simulink model "DT_SigmaDelta"  (Simulink 7.9)
settings: Solver=VariableStepDiscrete  StartTime=0.0  StopTime=1  RelTol=1e-6
PreLoadFcn:
  | load one_stage.mat
undefined symbols (not defined in the file or in its folder): DiscIntNeverNeededParam
libraries: dspmlti4 x21, simulink x3, dspvision x1
(part 1 of 13)
settings Model: Creator=abehbood  LastModifiedBy=Arnaldi Isacco
settings SolverCC: ConsecutiveZCsStepRelTol=128*eps  ZeroCrossControl=DisableAll
settings DataIOCC: LimitDataPoints=off  SaveFormat=StructureWithTime  SaveOutput=off  SaveTime=off
settings OptimizationCC: InitFltsAndDblsToZero=on
settings DebuggingCC: AlgebraicLoopMsg=none  SaveWithParameterizedLinksMsg=none  SignalResolutionControl=TryResolveAllWithWarning  FcnCallInpInsideContextMsg=Use local settings  StrictBusMsg=Warning
settings SFSimCC: SimParseCustomCode=off
settings GRTTargetCC: TargetFcnLib=ansi_tfl_tmw.mat  CombineOutputUpdateFcns=off  GRTInterface=on
settings ConfigurationSet: Description=SimMechanics 2G

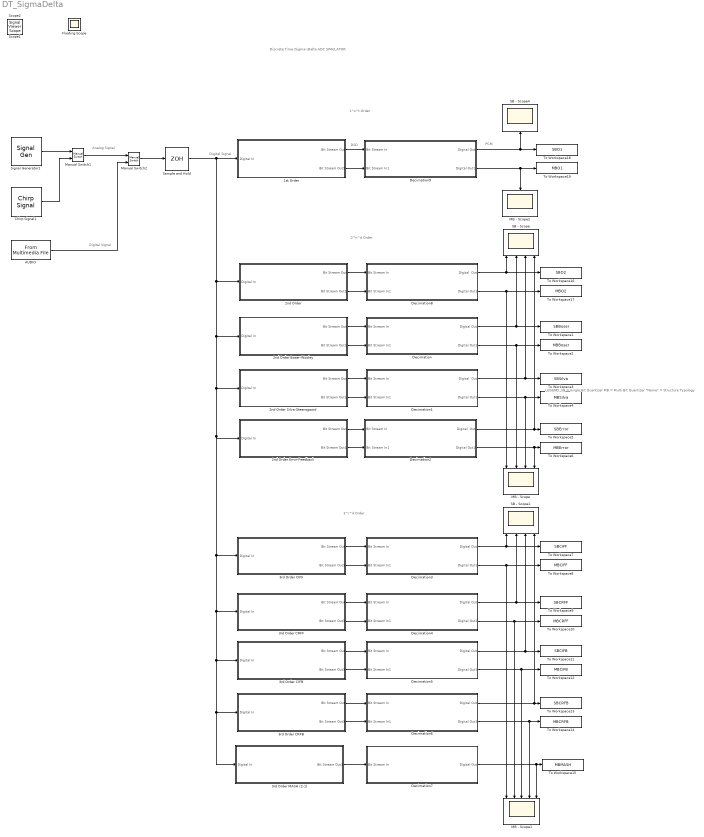
== system DT_SigmaDelta ==
  note: Discrete Time
      | \Sigma-\Delta ADC
      | SIMULATOR
  note: Digital Signal
  note: LEGEND:
      |
      | SB = Single Bit Quantizer
      |
      | MB = Multi Bit Quantizer
      |
      | "Name" = Structure Typology
  note: 2^n^d Order
  note: 3^r^d Order
  note: 1^s^t Order
  note: Analog Signal
  note: Digital Signal
  note: DSD
  note: PCM
  1st Order : Subsystem
  "2nd Order  " : Subsystem
  2nd Order Boser-Wooley : Subsystem
  2nd Order Error-Feedback : Subsystem
  "2nd Order Silva-Steensgaard " : Subsystem
  3rd Order CIFB : Subsystem
  3rd Order CIFF : Subsystem
  3rd Order CRFB : Subsystem
  3rd Order CRFF : Subsystem
  3rd Order MASH (2-1) : Subsystem
  AUDIO : dspvision/From Multimedia File  inputFilename=.\AudioSample.wav  loop=on  numPlays=inf  outputStreams=Audio only  videoDataType=single  audioDataType=double  inheritSampleTime=on  userDefinedSampleTime=1/30  noAudioOutput=off  isIntensityVideo=off  fourcc=RGB  colorVideoFormat=One multidimensional signal  outputEOF=off  dataOrg=Column-major  audioFrameSize=1  computeAudioFrameSize=off  outSamplingMode=Sample based
  Chirp Signal1 : simulink/Sources/Chirp Signal  f1=0.1  T=24/3000  f2=10000
  Decimation : Subsystem
  Decimation1 : Subsystem
  Decimation2 : Subsystem
  Decimation3 : Subsystem
  Decimation4 : Subsystem
  Decimation5 : Subsystem
  Decimation6 : Subsystem
  Decimation7 : Subsystem
  Decimation8 : Subsystem
  Decimation9 : Subsystem
  MB - Scope : Scope  NumInputPorts=4
      settings: TimeRange=0.008  YMin=-1.25~-1~-1~-5  YMax=1~1~1~5  SaveName=ScopeData2
  MB - Scope1 : Scope  NumInputPorts=5
      settings: TimeRange=0.008  YMin=-1.25~-1.25~-0.7~-0.75~-5  YMax=1.25~1.25~0.7~0.75~5  SaveName=ScopeData3
  MB - Scope2 : Scope
      settings: TimeRange=0.008  YMin=-1.25  YMax=1  SaveName=ScopeData6
  Manual Switch1 : simulink/Signal Routing/Manual Switch  sw=1  action=0  varsize=off
  Manual Switch2 : simulink/Signal Routing/Manual Switch  sw=1  action=0  varsize=off
  SB - Scope : Scope  NumInputPorts=4
      settings: TimeRange=0.008  YMin=-0.015~-0.01~-0.01~-0.015  YMax=0.015~0.0075~0.0125~0.015
  SB - Scope1 : Scope  NumInputPorts=4
      settings: TimeRange=0.008  YMin=-1.25~-0.8~-0.8~-0.75  YMax=1.25~0.8~0.8~0.75  SaveName=ScopeData4
  SB - Scope4 : Scope
      settings: TimeRange=0.008  YMin=-0.75  YMax=0.75  SaveName=ScopeData8
  Sample and Hold : ZeroOrderHold  SampleTime=1/(48e3*64)
  Signal Generator1 : SignalGenerator  Frequency=6283  Units=rad/sec
  To Workspace1 : ToWorkspace  VariableName=SBBoser  SampleTime=-1
  To Workspace10 : ToWorkspace  VariableName=MBCRFF  SampleTime=-1
  To Workspace11 : ToWorkspace  VariableName=SBCIFB  SampleTime=-1
  To Workspace12 : ToWorkspace  VariableName=MBCIFB  SampleTime=-1
  To Workspace13 : ToWorkspace  VariableName=SBCRFB  SampleTime=-1
  To Workspace14 : ToWorkspace  VariableName=MBCRFB  SampleTime=-1
  To Workspace15 : ToWorkspace  VariableName=MBMASH  SampleTime=-1
  To Workspace16 : ToWorkspace  VariableName=SBO2  SampleTime=-1
  To Workspace17 : ToWorkspace  VariableName=MBO2  SampleTime=-1
  To Workspace18 : ToWorkspace  VariableName=SBO1  SampleTime=-1
  To Workspace19 : ToWorkspace  VariableName=MBO1  SampleTime=-1
  To Workspace2 : ToWorkspace  VariableName=MBBoser  SampleTime=-1
  To Workspace3 : ToWorkspace  VariableName=SBSilva  SampleTime=-1
  To Workspace4 : ToWorkspace  VariableName=MBSilva  SampleTime=-1
  To Workspace5 : ToWorkspace  VariableName=SBError  SampleTime=-1
  To Workspace6 : ToWorkspace  VariableName=MBError  SampleTime=-1
  To Workspace7 : ToWorkspace  VariableName=SBCIFF  SampleTime=-1
  To Workspace8 : ToWorkspace  VariableName=MBCIFF  SampleTime=-1
  To Workspace9 : ToWorkspace  VariableName=SBCRFF  SampleTime=-1
  Floating Scope : Scope
      settings: Floating=on  YMin=-1  YMax=1
  Scope1 : SignalViewerScope  IOType=viewer  RefreshTime=0.035000
  Scope2 : SignalViewerScope  IOType=viewer  RefreshTime=0.035000
  wires:
  Decimation/1(Digital Out) -> To Workspace1/1, SB - Scope/2
  Decimation/2(Digital Out1) -> To Workspace2/1, MB - Scope/2
  Decimation1/1(Digital  Out) -> To Workspace3/1, SB - Scope/3
  Decimation1/2(Digital Out1) -> To Workspace4/1, MB - Scope/3
  Decimation2/1(Digital  Out) -> To Workspace5/1, SB - Scope/4
  Decimation2/2(Digital Out1) -> To Workspace6/1, MB - Scope/4
  Sample and Hold/1 -> 1st Order/1("Digital In "), "2nd Order  "/1(Digital In), 2nd Order Boser-Wooley/1("Digital In "), "2nd Order Silva-Steensgaard "/1(Digital In), 2nd Order Error-Feedback/1(Digital In), 3rd Order CIFB/1("Digital In "), 3rd Order CRFB/1("Digital In "), 3rd Order MASH (2-1)/1("Digital In "), 3rd Order CRFF/1(Digital In), 3rd Order CIFF/1(Digital In)
  2nd Order Boser-Wooley/2(Bit Stream Out1) -> Decimation/2(Bit Stream In1)
  2nd Order Boser-Wooley/1(Bit Stream Out) -> Decimation/1(Bit Stream In)
  "2nd Order Silva-Steensgaard "/1(Bit Stream Out) -> Decimation1/1(Bit Stream In)
  "2nd Order Silva-Steensgaard "/2(Bit Stream Out1) -> Decimation1/2(Bit Stream In1)
  2nd Order Error-Feedback/1(Bit Stream Out) -> Decimation2/1(Bit Stream In)
  2nd Order Error-Feedback/2(Bit Stream Out1) -> Decimation2/2(Bit Stream In1)
  Decimation6/1(Digital Out) -> To Workspace13/1, SB - Scope1/4
  Decimation6/2(Digital Out1) -> To Workspace14/1, MB - Scope1/4
  3rd Order CRFB/1(Bit Stream Out) -> Decimation6/1(Bit Stream In)
  3rd Order CRFB/2(Bit Stream Out1) -> Decimation6/2(Bit Stream In1)
  Decimation7/1(Digital Out) -> To Workspace15/1, MB - Scope1/5
  3rd Order MASH (2-1)/1(Bit Stream Out1) -> Decimation7/1(Bit Stream In)
  Decimation5/1(Digital Out) -> To Workspace11/1, SB - Scope1/3
  Decimation5/2(Digital Out1) -> To Workspace12/1, MB - Scope1/3
  Decimation4/1(Digital Out) -> To Workspace9/1, SB - Scope1/2
  Decimation4/2(Digital Out1) -> To Workspace10/1, MB - Scope1/2
  Decimation3/1(Digital Out) -> To Workspace7/1, SB - Scope1/1
  Decimation3/2(Digital Out1) -> To Workspace8/1, MB - Scope1/1
  3rd Order CIFF/1(Bit Stream Out) -> Decimation3/1(Bit Stream In)
  3rd Order CIFF/2(Bit Stream Out1) -> Decimation3/2(Bit Stream In1)
  3rd Order CIFB/1(Bit Stream Out) -> Decimation5/1(Bit Stream In)
  3rd Order CIFB/2(Bit Stream Out1) -> Decimation5/2(Bit Stream In1)
  "2nd Order  "/1(Bit Stream Out) -> Decimation8/1(Bit Stream In)
  "2nd Order  "/2(Bit Stream Out1) -> Decimation8/2(Bit Stream In1)
  Decimation8/1(Digital  Out) -> SB - Scope/1, To Workspace16/1
  Decimation8/2(Digital Out1) -> MB - Scope/1, To Workspace17/1
  Decimation9/1(Digital Out) -> To Workspace18/1, SB - Scope4/1
  1st Order/1(" Bit Stream Out") -> Decimation9/1(Bit Stream In)
  1st Order/2(" Bit Stream Out1") -> Decimation9/2(Bit Stream In1)
  Decimation9/2(Digital Out1) -> MB - Scope2/1, To Workspace19/1
  Signal Generator1/1 -> Manual Switch1/1
  Chirp Signal1/1 -> Manual Switch1/2
  Manual Switch1/1 -> Manual Switch2/1
  Manual Switch2/1 -> Sample and Hold/1
  AUDIO/1 -> Manual Switch2/2
  3rd Order CRFF/1(Bit Stream Out) -> Decimation4/1(Bit Stream In)
  3rd Order CRFF/2(Bit Stream Out1) -> Decimation4/2(Bit Stream In1)

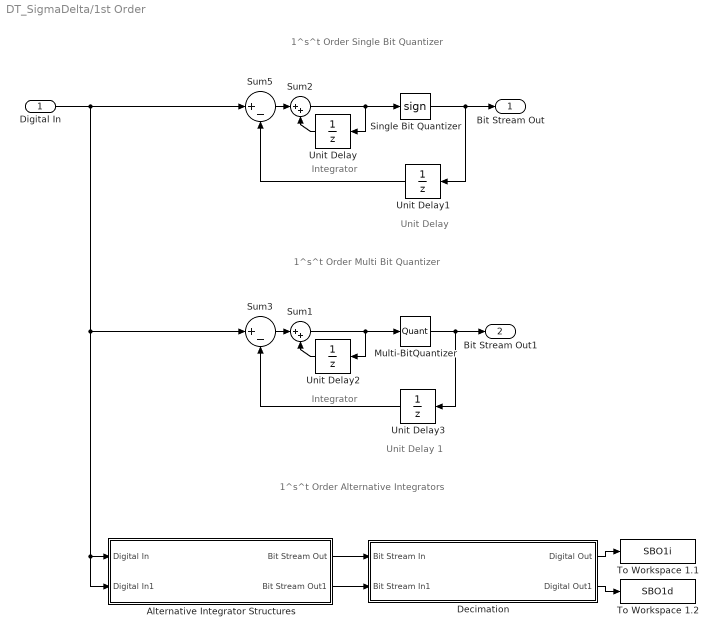
== system DT_SigmaDelta/1st Order ==
  note: 1^s^t Order Single Bit Quantizer
  note: 1^s^t Order Multi Bit Quantizer
  note: 1^s^t Order Alternative Integrators
  note: Integrator
  note: Integrator
  note: Unit Delay 1
  note: Unit Delay
  "Digital In " : Inport
  Alternative Integrator Structures : Subsystem
  Decimation : Subsystem
  Multi-BitQuantizer : Quantizer  QuantizationInterval=0.14  SampleTime=1/(48e3*64)
  Single Bit Quantizer : Signum  SampleTime=1/(48e3*64)
  Sum1 : Sum  Inputs=|++
  Sum2 : Sum  Inputs=|++
  Sum3 : Sum  Inputs=|+-  AccumDataTypeStr=double  SampleTime=1/(48e3*64)
  Sum5 : Sum  Inputs=|+-  AccumDataTypeStr=double  SampleTime=1/(48e3*64)
  To Workspace 1.1 : ToWorkspace  VariableName=SBO1i  SampleTime=-1
  To Workspace 1.2 : ToWorkspace  VariableName=SBO1d  SampleTime=-1
  Unit Delay{,1..3} (4 alike) : UnitDelay  SampleTime=1/(48e3*64)
  " Bit Stream Out" : Outport  OutDataTypeStr=double
  " Bit Stream Out1" : Outport  Port=2  OutDataTypeStr=double
  wires:
  "Digital In "/1 -> Sum5/1, Sum3/1, Alternative Integrator Structures/1(Digital In), Alternative Integrator Structures/2(Digital In1)
  Sum5/1 -> Sum2/1
  Unit Delay/1 -> Sum2/2
  Unit Delay1/1 -> Sum5/2
  Sum2/1 -> Unit Delay/1, Single Bit Quantizer/1
  Single Bit Quantizer/1 -> " Bit Stream Out"/1, Unit Delay1/1
  Sum3/1 -> Sum1/1
  Unit Delay2/1 -> Sum1/2
  Unit Delay3/1 -> Sum3/2
  Sum1/1 -> Unit Delay2/1, Multi-BitQuantizer/1
  Multi-BitQuantizer/1 -> Unit Delay3/1, " Bit Stream Out1"/1
  Decimation/1(Digital Out) -> To Workspace 1.1/1
  Alternative Integrator Structures/1(Bit Stream Out) -> Decimation/1(Bit Stream In)
  Alternative Integrator Structures/2(Bit Stream Out1) -> Decimation/2(Bit Stream In1)
  Decimation/2(Digital Out1) -> To Workspace 1.2/1

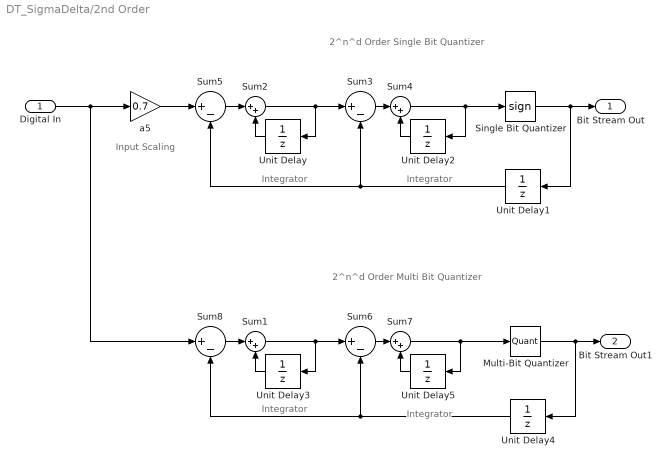
== system DT_SigmaDelta/2nd Order   ==
  note: 2^n^d Order Single Bit Quantizer
  note: 2^n^d Order Multi Bit Quantizer
  note: Input Scaling
  note: Integrator
  note: Integrator
  note: Integrator
  note: Integrator
  Digital In : Inport
  Multi-Bit Quantizer : Quantizer  QuantizationInterval=0.15  SampleTime=1/(48e3*64)
  Single Bit Quantizer : Signum  SampleTime=1/(48e3*64)
  Sum{1..2,4,7} (4 alike) : Sum  Inputs=|++  SampleTime=1/(48e3*64)
  Sum{3,5..6,8} (4 alike) : Sum  Inputs=|+-  AccumDataTypeStr=double  SampleTime=1/(48e3*64)
  Unit Delay{,1..5} (6 alike) : UnitDelay  SampleTime=1/(48e3*64)
  a5 : Gain  Gain=0.7  SampleTime=1/(48e3*64)
  Bit Stream Out : Outport  OutDataTypeStr=double
  Bit Stream Out1 : Outport  Port=2  OutDataTypeStr=double
  wires:
  Digital In/1 -> a5/1, Sum8/1
  Single Bit Quantizer/1 -> Bit Stream Out/1, Unit Delay1/1
  Multi-Bit Quantizer/1 -> Bit Stream Out1/1, Unit Delay4/1
  Sum8/1 -> Sum1/1
  Sum6/1 -> Sum7/1
  Unit Delay3/1 -> Sum1/2
  Sum1/1 -> Unit Delay3/1, Sum6/1
  Sum5/1 -> Sum2/1
  Unit Delay/1 -> Sum2/2
  Sum2/1 -> Sum3/1, Unit Delay/1
  Sum3/1 -> Sum4/1
  a5/1 -> Sum5/1
  Unit Delay2/1 -> Sum4/2
  Sum4/1 -> Unit Delay2/1, Single Bit Quantizer/1
  Unit Delay1/1 -> Sum5/2, Sum3/2
  Unit Delay5/1 -> Sum7/2
  Sum7/1 -> Unit Delay5/1, Multi-Bit Quantizer/1
  Unit Delay4/1 -> Sum8/2, Sum6/2

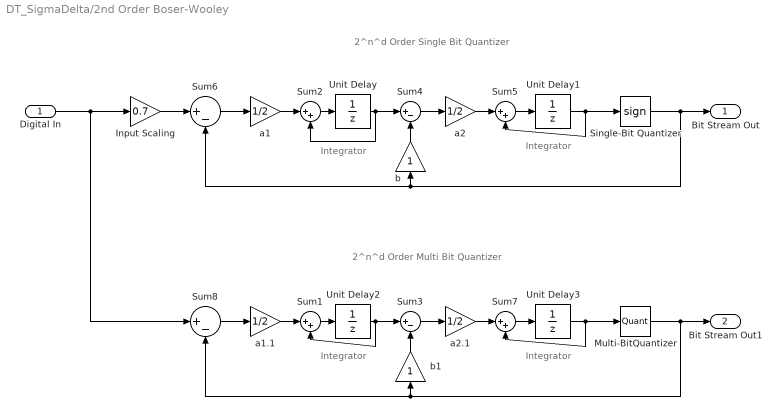
== system DT_SigmaDelta/2nd Order Boser-Wooley ==
  note: 2^n^d Order Single Bit Quantizer
  note: 2^n^d Order Multi Bit Quantizer
  note: Integrator
  note: Integrator
  note: Integrator
  note: Integrator
  "Digital In " : Inport
  Input Scaling : Gain  Gain=0.7  SampleTime=1/(48e3*64)
  Multi-BitQuantizer : Quantizer  QuantizationInterval=0.15  SampleTime=1/(48e3*64)
  Single-Bit Quantizer : Signum  SampleTime=1/(48e3*64)
  Sum{1..2,5,7} (4 alike) : Sum  Inputs=|++  SampleTime=1/(48e3*64)
  Sum3 : Sum  Inputs=|+-  SampleTime=1/(48e3*64)
  Sum4 : Sum  Inputs=|+-  SampleTime=1/(48e3*64)
  Sum6 : Sum  Inputs=|+-  AccumDataTypeStr=double  SampleTime=1/(48e3*64)
  Sum8 : Sum  Inputs=|+-  AccumDataTypeStr=double  SampleTime=1/(48e3*64)
  Unit Delay{,1..3} (4 alike) : UnitDelay  SampleTime=1/(48e3*64)
  a1 : Gain  Gain=1/2  SampleTime=1/(48e3*64)
  a1.1 : Gain  Gain=1/2  SampleTime=1/(48e3*64)
  a2 : Gain  Gain=1/2  SampleTime=1/(48e3*64)
  a2.1 : Gain  Gain=1/2  SampleTime=1/(48e3*64)
  b : Gain  SampleTime=1/(48e3*64)
  b1 : Gain  SampleTime=1/(48e3*64)
  Bit Stream Out : Outport  OutDataTypeStr=double
  Bit Stream Out1 : Outport  Port=2  OutDataTypeStr=double
  wires:
  "Digital In "/1 -> Input Scaling/1, Sum8/1
  Single-Bit Quantizer/1 -> b/1, Sum6/2, Bit Stream Out/1
  b/1 -> Sum4/2
  Sum5/1 -> Unit Delay1/1
  Sum6/1 -> a1/1
  Sum4/1 -> a2/1
  Unit Delay1/1 -> Single-Bit Quantizer/1, Sum5/2
  a2/1 -> Sum5/1
  a1/1 -> Sum2/1
  Unit Delay/1 -> Sum4/1, Sum2/2
  Sum2/1 -> Unit Delay/1
  Input Scaling/1 -> Sum6/1
  Multi-BitQuantizer/1 -> Bit Stream Out1/1, Sum8/2, b1/1
  b1/1 -> Sum3/2
  Sum7/1 -> Unit Delay3/1
  Sum8/1 -> a1.1/1
  Sum3/1 -> a2.1/1
  Unit Delay3/1 -> Sum7/2, Multi-BitQuantizer/1
  a2.1/1 -> Sum7/1
  a1.1/1 -> Sum1/1
  Unit Delay2/1 -> Sum1/2, Sum3/1
  Sum1/1 -> Unit Delay2/1

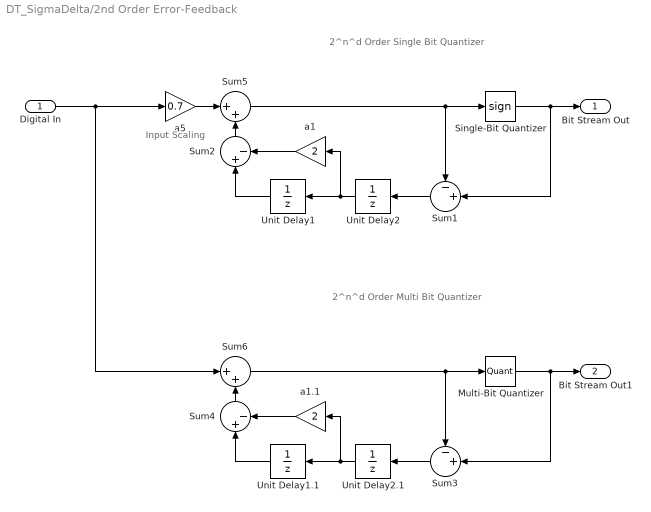
== system DT_SigmaDelta/2nd Order Error-Feedback ==
  note: Input Scaling
  note: 2^n^d Order Multi Bit Quantizer
  note: 2^n^d Order Single Bit Quantizer
  Digital In : Inport
  Multi-Bit Quantizer : Quantizer  QuantizationInterval=0.15  SampleTime=1/(48e3*64)
  Single-Bit Quantizer : Signum  SampleTime=1/(48e3*64)
  Sum1 : Sum  Inputs=-+|  AccumDataTypeStr=double  SampleTime=1/(48e3*64)
  Sum2 : Sum  Inputs=|+-  AccumDataTypeStr=double  SampleTime=1/(48e3*64)
  Sum3 : Sum  Inputs=-+|  AccumDataTypeStr=double  SampleTime=1/(48e3*64)
  Sum4 : Sum  Inputs=|+-  AccumDataTypeStr=double  SampleTime=1/(48e3*64)
  Sum5 : Sum  Inputs=|++  AccumDataTypeStr=double  SampleTime=1/(48e3*64)
  Sum6 : Sum  Inputs=|++  AccumDataTypeStr=double  SampleTime=1/(48e3*64)
  Unit Delay1 : UnitDelay  SampleTime=1/(48e3*64)
  Unit Delay1.1 : UnitDelay  SampleTime=1/(48e3*64)
  Unit Delay2 : UnitDelay  SampleTime=1/(48e3*64)
  Unit Delay2.1 : UnitDelay  SampleTime=1/(48e3*64)
  a1 : Gain  Gain=2  SampleTime=1/(48e3*64)
  a1.1 : Gain  Gain=2  SampleTime=1/(48e3*64)
  a5 : Gain  Gain=0.7  SampleTime=1/(48e3*64)
  Bit Stream Out : Outport  OutDataTypeStr=double
  Bit Stream Out1 : Outport  Port=2  OutDataTypeStr=double
  wires:
  Digital In/1 -> a5/1, Sum6/1
  Single-Bit Quantizer/1 -> Bit Stream Out/1, Sum1/2
  Unit Delay2/1 -> Unit Delay1/1, a1/1
  Unit Delay1/1 -> Sum2/1
  Sum2/1 -> Sum5/2
  a1/1 -> Sum2/2
  Sum5/1 -> Single-Bit Quantizer/1, Sum1/1
  Sum1/1 -> Unit Delay2/1
  a5/1 -> Sum5/1
  Multi-Bit Quantizer/1 -> Sum3/2, Bit Stream Out1/1
  Unit Delay2.1/1 -> a1.1/1, Unit Delay1.1/1
  Unit Delay1.1/1 -> Sum4/1
  Sum4/1 -> Sum6/2
  a1.1/1 -> Sum4/2
  Sum6/1 -> Sum3/1, Multi-Bit Quantizer/1
  Sum3/1 -> Unit Delay2.1/1

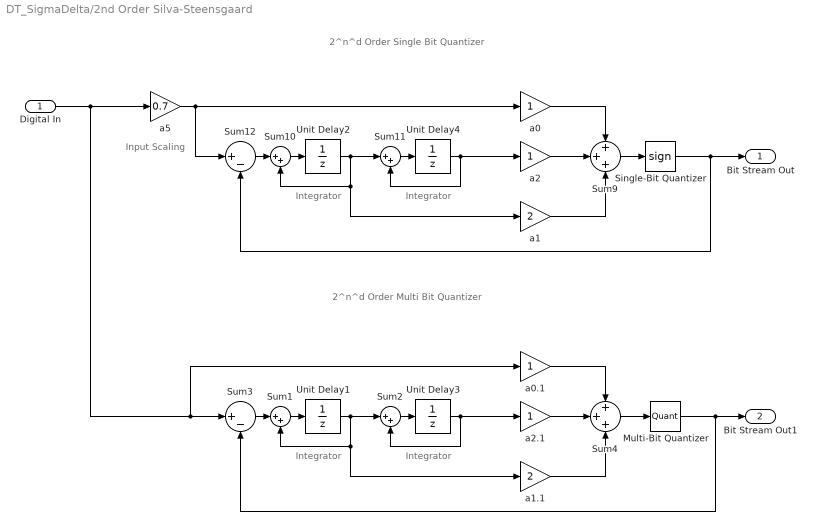
== system DT_SigmaDelta/2nd Order Silva-Steensgaard  ==
  note: 2^n^d Order Single Bit Quantizer
  note: 2^n^d Order Multi Bit Quantizer
  note: Input Scaling
  note: Integrator
  note: Integrator
  note: Integrator
  note: Integrator
  Digital In : Inport
  Multi-Bit Quantizer : Quantizer  QuantizationInterval=0.15  SampleTime=1/(48e3*64)
  Single-Bit Quantizer : Signum  SampleTime=1/(48e3*64)
  Sum{1..2,10..11} (4 alike) : Sum  Inputs=|++  SampleTime=1/(48e3*64)
  Sum12 : Sum  Inputs=|+-  AccumDataTypeStr=double  SampleTime=1/(48e3*64)
  Sum3 : Sum  Inputs=|+-  AccumDataTypeStr=double  SampleTime=1/(48e3*64)
  Sum4 : Sum  Inputs=+++  AccumDataTypeStr=double  SampleTime=1/(48e3*64)
  Sum9 : Sum  Inputs=+++  AccumDataTypeStr=double  SampleTime=1/(48e3*64)
  Unit Delay{1..4} (4 alike) : UnitDelay  SampleTime=1/(48e3*64)
  a0 : Gain  SampleTime=1/(48e3*64)
  a0.1 : Gain  SampleTime=1/(48e3*64)
  a1 : Gain  Gain=2  SampleTime=1/(48e3*64)
  a1.1 : Gain  Gain=2  SampleTime=1/(48e3*64)
  a2 : Gain  SampleTime=1/(48e3*64)
  a2.1 : Gain  SampleTime=1/(48e3*64)
  a5 : Gain  Gain=0.7  SampleTime=1/(48e3*64)
  Bit Stream Out : Outport  OutDataTypeStr=double
  Bit Stream Out1 : Outport  Port=2  OutDataTypeStr=double
  wires:
  Digital In/1 -> a5/1, Sum3/1, a0.1/1
  a5/1 -> a0/1, Sum12/1
  Unit Delay4/1 -> Sum11/2, a2/1
  Sum11/1 -> Unit Delay4/1
  Single-Bit Quantizer/1 -> Bit Stream Out/1, Sum12/2
  Sum12/1 -> Sum10/1
  Sum10/1 -> Unit Delay2/1
  Unit Delay2/1 -> Sum11/1, Sum10/2, a1/1
  a2/1 -> Sum9/2
  a0/1 -> Sum9/1
  a1/1 -> Sum9/3
  Sum9/1 -> Single-Bit Quantizer/1
  Unit Delay3/1 -> a2.1/1, Sum2/2
  Sum2/1 -> Unit Delay3/1
  Multi-Bit Quantizer/1 -> Sum3/2, Bit Stream Out1/1
  Sum3/1 -> Sum1/1
  Sum1/1 -> Unit Delay1/1
  Unit Delay1/1 -> a1.1/1, Sum1/2, Sum2/1
  a2.1/1 -> Sum4/2
  a0.1/1 -> Sum4/1
  a1.1/1 -> Sum4/3
  Sum4/1 -> Multi-Bit Quantizer/1

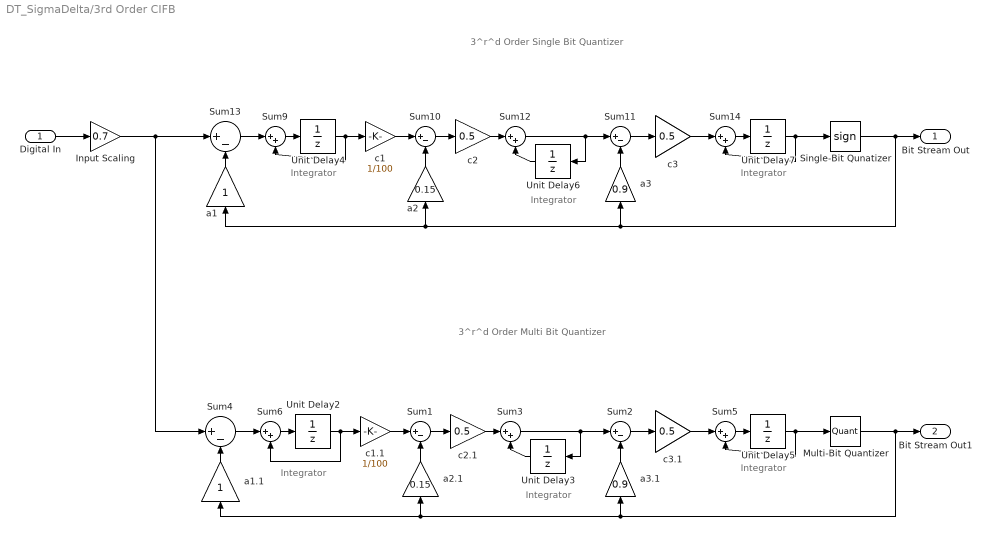
== system DT_SigmaDelta/3rd Order CIFB ==
  note: 3^r^d Order Single Bit Quantizer
  note: 3^r^d Order Multi Bit Quantizer
  note: Integrator
  note: Integrator
  note: Integrator
  note: Integrator
  note: Integrator
  note: Integrator
  "Digital In " : Inport
  Input Scaling : Gain  Gain=0.7  SampleTime=1/(48e3*64)
  Multi-Bit Quantizer : Quantizer  QuantizationInterval=0.15  SampleTime=1/(48e3*64)
  Single-Bit Qunatizer : Signum  SampleTime=1/(48e3*64)
  Sum{1..2,10..11} (4 alike) : Sum  Inputs=|+-
  Sum{3,5..6,9,12,14} (6 alike) : Sum  Inputs=|++  SampleTime=1/(48e3*64)
  Sum13 : Sum  Inputs=|+-  AccumDataTypeStr=double  SampleTime=1/(48e3*64)
  Sum4 : Sum  Inputs=|+-  AccumDataTypeStr=double  SampleTime=1/(48e3*64)
  Unit Delay{2..7} (6 alike) : UnitDelay  SampleTime=1/(48e3*64)
  a1 : Gain
  a1.1 : Gain
  a2 : Gain  Gain=0.15
  a2.1 : Gain  Gain=0.15
  a3 : Gain  Gain=0.9
  a3.1 : Gain  Gain=0.9
  c1 : Gain  Gain=1/100  SampleTime=1/(48e3*64)
  c1.1 : Gain  Gain=1/100  SampleTime=1/(48e3*64)
  c2 : Gain  Gain=0.5
  c2.1 : Gain  Gain=0.5
  c3 : Gain  Gain=0.5
  c3.1 : Gain  Gain=0.5
  Bit Stream Out : Outport  OutDataTypeStr=double
  Bit Stream Out1 : Outport  Port=2  OutDataTypeStr=double
  wires:
  c1/1 -> Sum10/1
  a2/1 -> Sum10/2
  "Digital In "/1 -> Input Scaling/1
  Single-Bit Qunatizer/1 -> a1/1, a2/1, a3/1, Bit Stream Out/1
  a3/1 -> Sum11/2
  a1/1 -> Sum13/2
  Sum13/1 -> Sum9/1
  Sum11/1 -> c3/1
  Sum10/1 -> c2/1
  Unit Delay6/1 -> Sum12/2
  Sum12/1 -> Sum11/1, Unit Delay6/1
  c2/1 -> Sum12/1
  c3/1 -> Sum14/1
  Input Scaling/1 -> Sum4/1, Sum13/1
  Multi-Bit Quantizer/1 -> a3.1/1, a2.1/1, a1.1/1, Bit Stream Out1/1
  a3.1/1 -> Sum2/2
  a1.1/1 -> Sum4/2
  Sum4/1 -> Sum6/1
  Sum2/1 -> c3.1/1
  Sum1/1 -> c2.1/1
  a2.1/1 -> Sum1/2
  c1.1/1 -> Sum1/1
  Unit Delay3/1 -> Sum3/2
  Sum3/1 -> Sum2/1, Unit Delay3/1
  c2.1/1 -> Sum3/1
  c3.1/1 -> Sum5/1
  Sum9/1 -> Unit Delay4/1
  Unit Delay4/1 -> Sum9/2, c1/1
  Sum14/1 -> Unit Delay7/1
  Unit Delay7/1 -> Single-Bit Qunatizer/1, Sum14/2
  Sum5/1 -> Unit Delay5/1
  Unit Delay5/1 -> Multi-Bit Quantizer/1, Sum5/2
  Sum6/1 -> Unit Delay2/1
  Unit Delay2/1 -> c1.1/1, Sum6/2

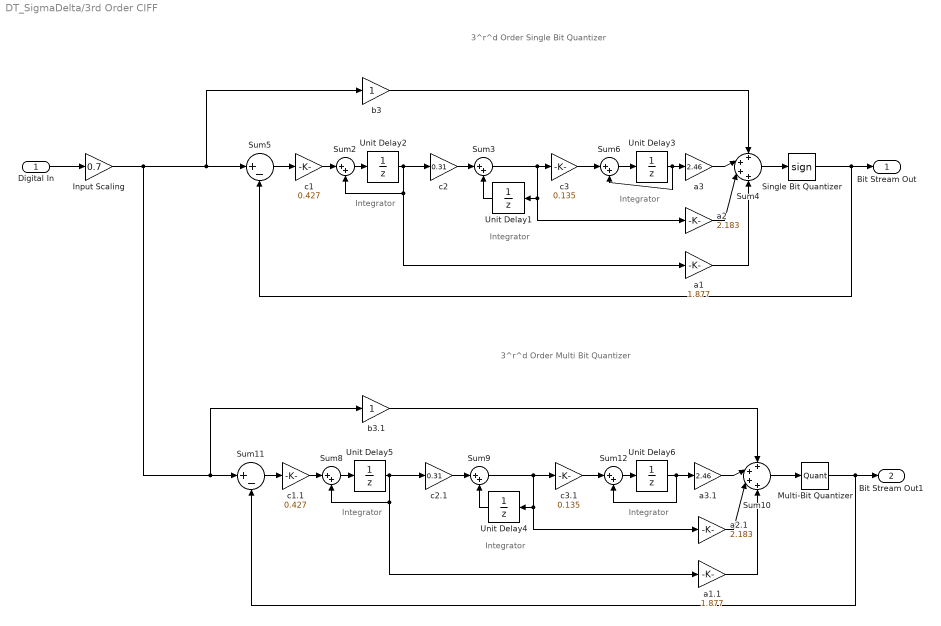
== system DT_SigmaDelta/3rd Order CIFF ==
  note: Integrator
  note: Integrator
  note: Integrator
  note: Integrator
  note: Integrator
  note: Integrator
  note: 3^r^d Order Multi Bit Quantizer
  note: 3^r^d Order Single Bit Quantizer
  Digital In : Inport
  Input Scaling : Gain  Gain=0.7  SampleTime=1/(48e3*64)
  Multi-Bit Quantizer : Quantizer  QuantizationInterval=0.125  SampleTime=1/(48e3*64)
  Single Bit Quantizer : Signum  SampleTime=1/(48e3*64)
  Sum10 : Sum  Inputs=++++  AccumDataTypeStr=double  SampleTime=1/(48e3*64)
  Sum11 : Sum  Inputs=|+-  AccumDataTypeStr=double  SampleTime=1/(48e3*64)
  Sum{2..3,6,8..9,12} (6 alike) : Sum  Inputs=|++  SampleTime=1/(48e3*64)
  Sum4 : Sum  Inputs=++++  AccumDataTypeStr=double  SampleTime=1/(48e3*64)
  Sum5 : Sum  Inputs=|+-  AccumDataTypeStr=double  SampleTime=1/(48e3*64)
  Unit Delay{1..6} (6 alike) : UnitDelay  SampleTime=1/(48e3*64)
  a1 : Gain  Gain=1.877  SampleTime=1/(48e3*64)
  a1.1 : Gain  Gain=1.877  SampleTime=1/(48e3*64)
  a2 : Gain  Gain=2.183  SampleTime=1/(48e3*64)
  a2.1 : Gain  Gain=2.183  SampleTime=1/(48e3*64)
  a3 : Gain  Gain=2.46  SampleTime=1/(48e3*64)
  a3.1 : Gain  Gain=2.46  SampleTime=1/(48e3*64)
  b3 : Gain  SampleTime=1/(48e3*64)
  b3.1 : Gain  SampleTime=1/(48e3*64)
  c1 : Gain  Gain=0.427  SampleTime=1/(48e3*64)
  c1.1 : Gain  Gain=0.427  SampleTime=1/(48e3*64)
  c2 : Gain  Gain=0.31  SampleTime=1/(48e3*64)
  c2.1 : Gain  Gain=0.31  SampleTime=1/(48e3*64)
  c3 : Gain  Gain=0.135  SampleTime=1/(48e3*64)
  c3.1 : Gain  Gain=0.135  SampleTime=1/(48e3*64)
  Bit Stream Out : Outport  OutDataTypeStr=double
  Bit Stream Out1 : Outport  Port=2  OutDataTypeStr=double
  wires:
  Sum6/1 -> Unit Delay3/1
  Unit Delay3/1 -> Sum6/2, a3/1
  Sum3/1 -> Unit Delay1/1, a2/1, c3/1
  Unit Delay1/1 -> Sum3/2
  Unit Delay6/1 -> Sum12/2, a3.1/1
  Sum12/1 -> Unit Delay6/1
  Unit Delay5/1 -> a1.1/1, Sum8/2, c2.1/1
  Sum8/1 -> Unit Delay5/1
  Unit Delay2/1 -> a1/1, Sum2/2, c2/1
  Sum2/1 -> Unit Delay2/1
  Input Scaling/1 -> b3.1/1, Sum11/1, b3/1, Sum5/1
  b3.1/1 -> Sum10/1
  b3/1 -> Sum4/1
  Sum10/1 -> Multi-Bit Quantizer/1
  Unit Delay4/1 -> Sum9/2
  Sum9/1 -> c3.1/1, a2.1/1, Unit Delay4/1
  a3.1/1 -> Sum10/2
  a1.1/1 -> Sum10/4
  c3.1/1 -> Sum12/1
  c2.1/1 -> Sum9/1
  c1.1/1 -> Sum8/1
  Sum11/1 -> c1.1/1
  Multi-Bit Quantizer/1 -> Sum11/2, Bit Stream Out1/1
  a2.1/1 -> Sum10/3
  Sum4/1 -> Single Bit Quantizer/1
  a3/1 -> Sum4/2
  a1/1 -> Sum4/4
  c3/1 -> Sum6/1
  c2/1 -> Sum3/1
  c1/1 -> Sum2/1
  Sum5/1 -> c1/1
  Single Bit Quantizer/1 -> Sum5/2, Bit Stream Out/1
  Digital In/1 -> Input Scaling/1
  a2/1 -> Sum4/3

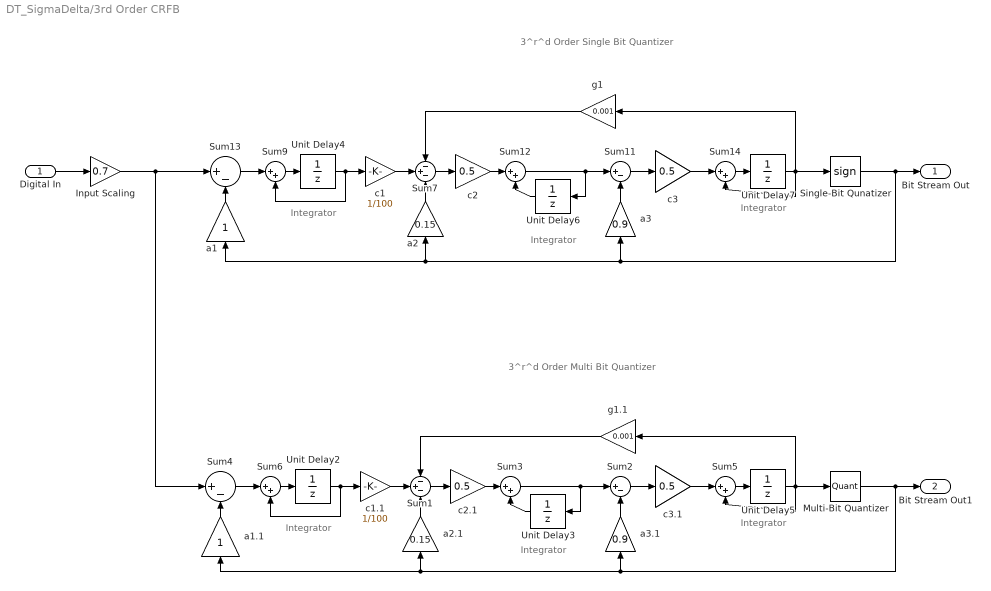
== system DT_SigmaDelta/3rd Order CRFB ==
  note: 3^r^d Order Multi Bit Quantizer
  note: 3^r^d Order Single Bit Quantizer
  note: Integrator
  note: Integrator
  note: Integrator
  note: Integrator
  note: Integrator
  note: Integrator
  "Digital In " : Inport
  Input Scaling : Gain  Gain=0.7  SampleTime=1/(48e3*64)
  Multi-Bit Quantizer : Quantizer  QuantizationInterval=0.125  SampleTime=1/(48e3*64)
  Single-Bit Qunatizer : Signum  SampleTime=1/(48e3*64)
  Sum1 : Sum  Inputs=-+-
  Sum11 : Sum  Inputs=|+-
  Sum{3,5..6,9,12,14} (6 alike) : Sum  Inputs=|++  SampleTime=1/(48e3*64)
  Sum13 : Sum  Inputs=|+-  AccumDataTypeStr=double  SampleTime=1/(48e3*64)
  Sum2 : Sum  Inputs=|+-
  Sum4 : Sum  Inputs=|+-  AccumDataTypeStr=double  SampleTime=1/(48e3*64)
  Sum7 : Sum  Inputs=-+-
  Unit Delay{2..7} (6 alike) : UnitDelay  SampleTime=1/(48e3*64)
  a1 : Gain
  a1.1 : Gain
  a2 : Gain  Gain=0.15
  a2.1 : Gain  Gain=0.15
  a3 : Gain  Gain=0.9
  a3.1 : Gain  Gain=0.9
  c1 : Gain  Gain=1/100  SampleTime=1/(48e3*64)
  c1.1 : Gain  Gain=1/100  SampleTime=1/(48e3*64)
  c2 : Gain  Gain=0.5
  c2.1 : Gain  Gain=0.5
  c3 : Gain  Gain=0.5
  c3.1 : Gain  Gain=0.5
  g1 : Gain  Gain=0.001
  g1.1 : Gain  Gain=0.001
  Bit Stream Out : Outport  OutDataTypeStr=double
  Bit Stream Out1 : Outport  Port=2  OutDataTypeStr=double
  wires:
  Unit Delay2/1 -> Sum6/2, c1.1/1
  Sum6/1 -> Unit Delay2/1
  Unit Delay5/1 -> Sum5/2, Multi-Bit Quantizer/1, g1.1/1
  Sum5/1 -> Unit Delay5/1
  Unit Delay7/1 -> Sum14/2, Single-Bit Qunatizer/1, g1/1
  Sum14/1 -> Unit Delay7/1
  Unit Delay4/1 -> c1/1, Sum9/2
  Sum9/1 -> Unit Delay4/1
  c3.1/1 -> Sum5/1
  c2.1/1 -> Sum3/1
  Sum3/1 -> Unit Delay3/1, Sum2/1
  Unit Delay3/1 -> Sum3/2
  c1.1/1 -> Sum1/2
  a2.1/1 -> Sum1/3
  Sum1/1 -> c2.1/1
  Sum2/1 -> c3.1/1
  Sum4/1 -> Sum6/1
  a1.1/1 -> Sum4/2
  a3.1/1 -> Sum2/2
  Multi-Bit Quantizer/1 -> Bit Stream Out1/1, a1.1/1, a2.1/1, a3.1/1
  Input Scaling/1 -> Sum13/1, Sum4/1
  c3/1 -> Sum14/1
  c2/1 -> Sum12/1
  Sum12/1 -> Unit Delay6/1, Sum11/1
  Unit Delay6/1 -> Sum12/2
  Sum7/1 -> c2/1
  Sum11/1 -> c3/1
  Sum13/1 -> Sum9/1
  a1/1 -> Sum13/2
  a3/1 -> Sum11/2
  Single-Bit Qunatizer/1 -> Bit Stream Out/1, a3/1, a2/1, a1/1
  "Digital In "/1 -> Input Scaling/1
  a2/1 -> Sum7/3
  c1/1 -> Sum7/2
  g1/1 -> Sum7/1
  g1.1/1 -> Sum1/1

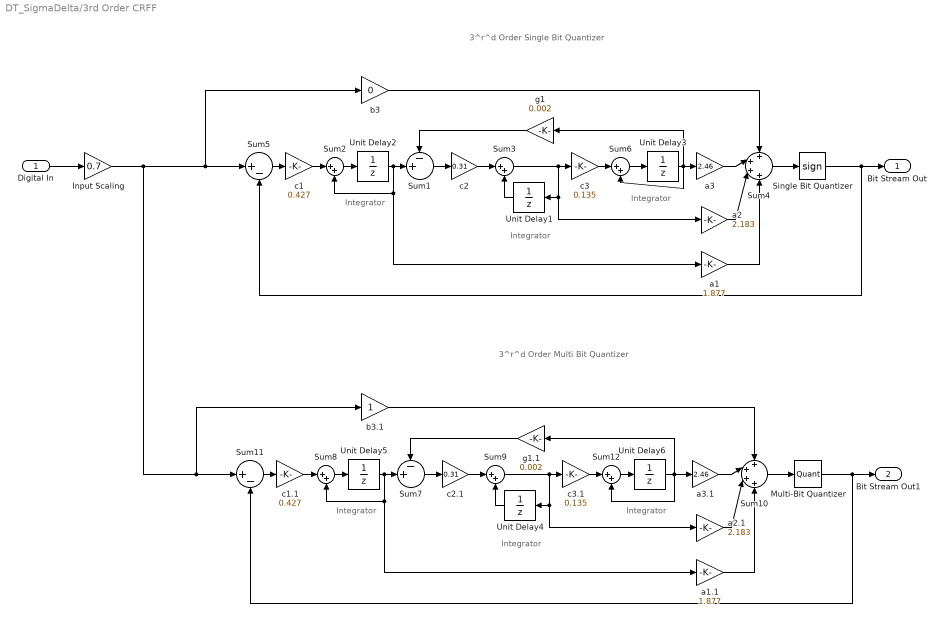
== system DT_SigmaDelta/3rd Order CRFF ==
  note: 3^r^d Order Single Bit Quantizer
  note: 3^r^d Order Multi Bit Quantizer
  note: Integrator
  note: Integrator
  note: Integrator
  note: Integrator
  note: Integrator
  note: Integrator
  Digital In : Inport
  Input Scaling : Gain  Gain=0.7  SampleTime=1/(48e3*64)
  Multi-Bit Quantizer : Quantizer  QuantizationInterval=0.125  SampleTime=1/(48e3*64)
  Single Bit Quantizer : Signum  SampleTime=1/(48e3*64)
  Sum1 : Sum  Inputs=-+|  AccumDataTypeStr=double  SampleTime=1/(48e3*64)
  Sum10 : Sum  Inputs=++++  AccumDataTypeStr=double  SampleTime=1/(48e3*64)
  Sum11 : Sum  Inputs=|+-  AccumDataTypeStr=double  SampleTime=1/(48e3*64)
  Sum{2..3,6,8..9,12} (6 alike) : Sum  Inputs=|++  SampleTime=1/(48e3*64)
  Sum4 : Sum  Inputs=++++  AccumDataTypeStr=double  SampleTime=1/(48e3*64)
  Sum5 : Sum  Inputs=|+-  AccumDataTypeStr=double  SampleTime=1/(48e3*64)
  Sum7 : Sum  Inputs=-+|  AccumDataTypeStr=double  SampleTime=1/(48e3*64)
  Unit Delay{1..6} (6 alike) : UnitDelay  SampleTime=1/(48e3*64)
  a1 : Gain  Gain=1.877  SampleTime=1/(48e3*64)
  a1.1 : Gain  Gain=1.877  SampleTime=1/(48e3*64)
  a2 : Gain  Gain=2.183  SampleTime=1/(48e3*64)
  a2.1 : Gain  Gain=2.183  SampleTime=1/(48e3*64)
  a3 : Gain  Gain=2.46  SampleTime=1/(48e3*64)
  a3.1 : Gain  Gain=2.46  SampleTime=1/(48e3*64)
  b3 : Gain  Gain=0  SampleTime=1/(48e3*64)
  b3.1 : Gain  SampleTime=1/(48e3*64)
  c1 : Gain  Gain=0.427  SampleTime=1/(48e3*64)
  c1.1 : Gain  Gain=0.427  SampleTime=1/(48e3*64)
  c2 : Gain  Gain=0.31  SampleTime=1/(48e3*64)
  c2.1 : Gain  Gain=0.31  SampleTime=1/(48e3*64)
  c3 : Gain  Gain=0.135  SampleTime=1/(48e3*64)
  c3.1 : Gain  Gain=0.135  SampleTime=1/(48e3*64)
  g1 : Gain  Gain=0.002  SampleTime=1/(48e3*64)
  g1.1 : Gain  Gain=0.002  SampleTime=1/(48e3*64)
  Bit Stream Out : Outport  OutDataTypeStr=double
  Bit Stream Out1 : Outport  Port=2  OutDataTypeStr=double
  wires:
  a2/1 -> Sum4/3
  Digital In/1 -> Input Scaling/1
  Single Bit Quantizer/1 -> Bit Stream Out/1, Sum5/2
  Sum5/1 -> c1/1
  Sum1/1 -> c2/1
  c1/1 -> Sum2/1
  c2/1 -> Sum3/1
  c3/1 -> Sum6/1
  a1/1 -> Sum4/4
  a3/1 -> Sum4/2
  g1/1 -> Sum1/1
  Sum4/1 -> Single Bit Quantizer/1
  a2.1/1 -> Sum10/3
  Multi-Bit Quantizer/1 -> Bit Stream Out1/1, Sum11/2
  Sum11/1 -> c1.1/1
  Sum7/1 -> c2.1/1
  c1.1/1 -> Sum8/1
  c2.1/1 -> Sum9/1
  c3.1/1 -> Sum12/1
  a1.1/1 -> Sum10/4
  a3.1/1 -> Sum10/2
  Sum9/1 -> Unit Delay4/1, a2.1/1, c3.1/1
  Unit Delay4/1 -> Sum9/2
  g1.1/1 -> Sum7/1
  Sum10/1 -> Multi-Bit Quantizer/1
  b3/1 -> Sum4/1
  b3.1/1 -> Sum10/1
  Input Scaling/1 -> Sum5/1, b3/1, Sum11/1, b3.1/1
  Sum2/1 -> Unit Delay2/1
  Unit Delay2/1 -> Sum1/2, Sum2/2, a1/1
  Sum8/1 -> Unit Delay5/1
  Unit Delay5/1 -> Sum7/2, Sum8/2, a1.1/1
  Sum12/1 -> Unit Delay6/1
  Unit Delay6/1 -> g1.1/1, a3.1/1, Sum12/2
  Unit Delay1/1 -> Sum3/2
  Sum3/1 -> c3/1, a2/1, Unit Delay1/1
  Unit Delay3/1 -> g1/1, a3/1, Sum6/2
  Sum6/1 -> Unit Delay3/1

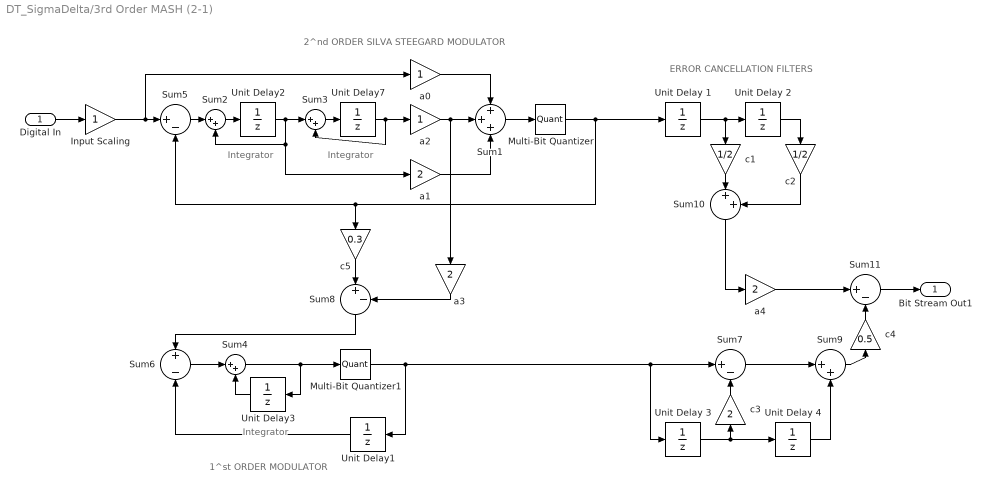
== system DT_SigmaDelta/3rd Order MASH (2-1) ==
  note: 1^st ORDER MODULATOR
  note: 2^nd ORDER SILVA STEEGARD MODULATOR
  note: ERROR CANCELLATION FILTERS
  note: Integrator
  note: Integrator
  note: Integrator
  "Digital In " : Inport
  Input Scaling : Gain  SampleTime=1/(48e3*64)
  Multi-Bit Quantizer : Quantizer  QuantizationInterval=0.125  SampleTime=1/(48e3*64)
  Multi-Bit Quantizer1 : Quantizer  QuantizationInterval=0.125  SampleTime=1/(48e3*64)
  Sum1 : Sum  Inputs=+++  AccumDataTypeStr=double  SampleTime=1/(48e3*64)
  Sum10 : Sum  Inputs=|++  AccumDataTypeStr=double  SampleTime=1/(48e3*64)
  Sum{5,7..8,11} (4 alike) : Sum  Inputs=|+-  AccumDataTypeStr=double  SampleTime=1/(48e3*64)
  Sum2 : Sum  Inputs=|++  SampleTime=1/(48e3*64)
  Sum3 : Sum  Inputs=|++  SampleTime=1/(48e3*64)
  Sum4 : Sum  Inputs=|++  SampleTime=1/(48e3*64)
  Sum6 : Sum  Inputs=+-  AccumDataTypeStr=double  SampleTime=1/(48e3*64)
  Sum9 : Sum  Inputs=|++  AccumDataTypeStr=double  SampleTime=1/(48e3*64)
  Unit Delay {1..4} (4 alike) : UnitDelay  SampleTime=1/(48e3*64)
  Unit Delay{1..3,7} (4 alike) : UnitDelay  SampleTime=1/(48e3*64)
  a0 : Gain  SampleTime=1/(48e3*64)
  a1 : Gain  Gain=2  SampleTime=1/(48e3*64)
  a2 : Gain  SampleTime=1/(48e3*64)
  a3 : Gain  Gain=2  SampleTime=1/(48e3*64)
  a4 : Gain  Gain=2  SampleTime=1/(48e3*64)
  c1 : Gain  Gain=1/2  SampleTime=1/(48e3*64)
  c2 : Gain  Gain=1/2  SampleTime=1/(48e3*64)
  c3 : Gain  Gain=2  SampleTime=1/(48e3*64)
  c4 : Gain  Gain=0.5  SampleTime=1/(48e3*64)
  c5 : Gain  Gain=0.3  SampleTime=1/(48e3*64)
  Bit Stream Out1 : Outport  OutDataTypeStr=double
  wires:
  Input Scaling/1 -> Sum5/1, a0/1
  "Digital In "/1 -> Input Scaling/1
  Multi-Bit Quantizer1/1 -> Sum7/1, Unit Delay 3/1, Unit Delay1/1
  Sum7/1 -> Sum9/1
  Unit Delay 3/1 -> Unit Delay 4/1, c3/1
  Unit Delay 4/1 -> Sum9/2
  c3/1 -> Sum7/2
  Unit Delay 1/1 -> Unit Delay 2/1, c1/1
  Unit Delay 2/1 -> c2/1
  c1/1 -> Sum10/1
  c2/1 -> Sum10/2
  Sum11/1 -> Bit Stream Out1/1
  Unit Delay7/1 -> a2/1, Sum3/2
  Sum3/1 -> Unit Delay7/1
  Multi-Bit Quantizer/1 -> Unit Delay 1/1, Sum5/2, c5/1
  Sum5/1 -> Sum2/1
  Sum2/1 -> Unit Delay2/1
  Unit Delay2/1 -> Sum3/1, Sum2/2, a1/1
  a2/1 -> Sum1/2, a3/1
  a0/1 -> Sum1/1
  a1/1 -> Sum1/3
  Sum1/1 -> Multi-Bit Quantizer/1
  Sum9/1 -> c4/1
  a3/1 -> Sum8/2
  Sum6/1 -> Sum4/1
  c4/1 -> Sum11/2
  Sum8/1 -> Sum6/1
  Sum10/1 -> a4/1
  a4/1 -> Sum11/1
  c5/1 -> Sum8/1
  Unit Delay3/1 -> Sum4/2
  Sum4/1 -> Multi-Bit Quantizer1/1, Unit Delay3/1
  Unit Delay1/1 -> Sum6/2
